simulink library "ODEHubs_components"  (R2020b)
settings: Solver=VariableStepAuto  StartTime=0.0  StopTime=10.0  RelTol=1e-3
values from neighbouring files (symbols this model uses):
  I = aux    [EH_definition_Simulink.m]
  O = aux    [EH_definition_Simulink.m]
undefined symbols (not defined in the file or in its folder): AbsorptionChiller, beta1, BiomassBoiler, Boiler, CN0, CombinedHeatAndPower, cpa, DesalinationPlant, dispatch_factor, DN0, efficiency, HeatPump, IrrigationPump, Low, Low1, Low2, Max_in, Max_out, Min_in, NanofiltrationPlant, PVModules, r_c, r_d, ReversibleHeatPump, SolarCollector, StorageSystem, T_muestreo, Tm, Up, Up1, Up2
(part 2 of 2)

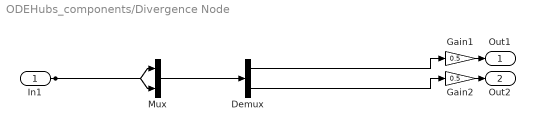
== system ODEHubs_components/Divergence Node ==
  In1 : Inport
  Demux : Demux  Outputs=2
  Gain1 : Gain  Gain=0.5
  Gain2 : Gain  Gain=0.5
  Mux : Mux  Inputs=2
  Out1 : Outport
  Out2 : Outport  Port=2
  wires:
  In1/1 -> Mux/1, Mux/2
  Demux/1 -> Gain1/1
  Gain1/1 -> Out1/1
  Demux/2 -> Gain2/1
  Gain2/1 -> Out2/1
  Mux/1 -> Demux/1

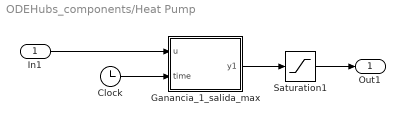
== system ODEHubs_components/Heat Pump ==
  In1 : Inport
  Clock : Clock
  Ganancia_1_salida_max : MATLAB Function  TreatAsAtomicUnit=on  mask{Max_in=10, efficiency=[5.4], T_muestreo=T_muestreo, dispatch_factor=1}
      mask prompts: Max_in "Máximo"; efficiency "Eficiencia"; T_muestreo "Tiempo de muestreo"; dispatch_factor "Coeficiente de reparto"
  Saturation1 : Saturate  UpperLimit=Max_out(1)  LowerLimit=-inf
  Out1 : Outport  VectorParamsAs1DForOutWhenUnconnected=off
  wires:
  Saturation1/1 -> Out1/1
  Clock/1 -> Ganancia_1_salida_max/2(time)
  In1/1 -> Ganancia_1_salida_max/1(u)
  Ganancia_1_salida_max/1(y1) -> Saturation1/1

== system ODEHubs_components/Input ==
  Input : FromWorkspace  VariableName=simin
  Out1 : Outport
  wires:
  Input/1 -> Out1/1

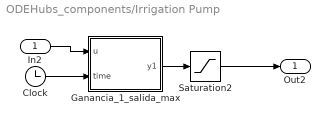
== system ODEHubs_components/Irrigation Pump ==
  In2 : Inport
  Clock : Clock
  Ganancia_1_salida_max : MATLAB Function  TreatAsAtomicUnit=on  mask{Max_in=150, efficiency=1, T_muestreo=T_muestreo, dispatch_factor=beta1}
      mask prompts: Max_in "Máximo"; efficiency "Eficiencia"; T_muestreo "Tiempo de muestreo"; dispatch_factor "Coeficiente de reparto"
  Saturation2 : Saturate  UpperLimit=Max_out  LowerLimit=-inf
  Out2 : Outport  VectorParamsAs1DForOutWhenUnconnected=off
  wires:
  Clock/1 -> Ganancia_1_salida_max/2(time)
  Saturation2/1 -> Out2/1
  In2/1 -> Ganancia_1_salida_max/1(u)
  Ganancia_1_salida_max/1(y1) -> Saturation2/1

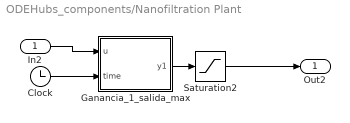
== system ODEHubs_components/Nanofiltration Plant ==
  In2 : Inport
  Clock : Clock
  Ganancia_1_salida_max : MATLAB Function  TreatAsAtomicUnit=on  mask{Max_in=Max_in, efficiency=efficiency, T_muestreo=T_muestreo, dispatch_factor=beta1}
      mask prompts: Max_in "Máximo"; efficiency "Eficiencia"; T_muestreo "Tiempo de muestreo"; dispatch_factor "Coeficiente de reparto"
  Saturation2 : Saturate  UpperLimit=Max_out  LowerLimit=-inf
  Out2 : Outport  VectorParamsAs1DForOutWhenUnconnected=off
  wires:
  Ganancia_1_salida_max/1(y1) -> Saturation2/1
  Saturation2/1 -> Out2/1
  In2/1 -> Ganancia_1_salida_max/1(u)
  Clock/1 -> Ganancia_1_salida_max/2(time)

== system ODEHubs_components/Output ==
  In1 : Inport
  Market Sales : Constant  Value=0
  Output : ToWorkspace  VariableName=simout  SaveFormat=Timeseries  SampleTime=-1
  Sum : Sum  Inputs=-+|
  wires:
  In1/1 -> Sum/2
  Sum/1 -> Output/1
  Market Sales/1 -> Sum/1

== system ODEHubs_components/PV Modules ==
  In1 : Inport
  Clock : Clock
  Ganancia_1_salida_max : MATLAB Function  TreatAsAtomicUnit=on  mask{Max_in=1200, efficiency=[0.211], T_muestreo=T_muestreo, dispatch_factor=1}
      mask prompts: Max_in "Máximo"; efficiency "Eficiencia"; T_muestreo "Tiempo de muestreo"; dispatch_factor "Coeficiente de reparto"
  Saturation1 : Saturate  UpperLimit=Max_out  LowerLimit=-inf
  Out1 : Outport  VectorParamsAs1DForOutWhenUnconnected=off
  wires:
  Saturation1/1 -> Out1/1
  Ganancia_1_salida_max/1(y1) -> Saturation1/1
  In1/1 -> Ganancia_1_salida_max/1(u)
  Clock/1 -> Ganancia_1_salida_max/2(time)

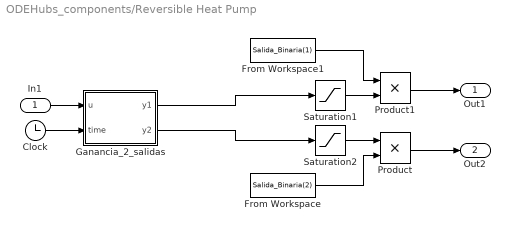
== system ODEHubs_components/Reversible Heat Pump ==
  In1 : Inport
  Clock : Clock
  From Workspace : FromWorkspace  VariableName=Salida_Binaria(2)
  From Workspace1 : FromWorkspace  VariableName=Salida_Binaria(1)
  Ganancia_2_salidas : MATLAB Function  TreatAsAtomicUnit=on  mask{efficiency=efficiency, T_muestreo=T_muestreo, Max_in=Max_in, Min_in=Min_in, dispatch_factor=1}
      mask prompts: efficiency "Eficiencia"; T_muestreo "Tiempo de muestreo"; Max_in "Entrada máxima"; Min_in "Entrada mínima"; dispatch_factor "Coeficiente de reparto"
  Product : Product
  Product1 : Product
  Saturation1 : Saturate  UpperLimit=Max_out(1)  LowerLimit=-inf
  Saturation2 : Saturate  UpperLimit=Max_out(2)  LowerLimit=-inf
  Out1 : Outport  VectorParamsAs1DForOutWhenUnconnected=off
  Out2 : Outport  Port=2  VectorParamsAs1DForOutWhenUnconnected=off
  wires:
  In1/1 -> Ganancia_2_salidas/1(u)
  Clock/1 -> Ganancia_2_salidas/2(time)
  Ganancia_2_salidas/1(y1) -> Saturation1/1
  Ganancia_2_salidas/2(y2) -> Saturation2/1
  Product/1 -> Out2/1
  Saturation2/1 -> Product/1
  Saturation1/1 -> Product1/2
  Product1/1 -> Out1/1
  From Workspace/1 -> Product/2
  From Workspace1/1 -> Product1/1

== system ODEHubs_components/Solar Collector ==
  In1 : Inport
  Clock : Clock
  Ganancia_1_salida_max : MATLAB Function  TreatAsAtomicUnit=on  mask{Max_in=1200, efficiency=[0.211], T_muestreo=T_muestreo, dispatch_factor=1}
      mask prompts: Max_in "Máximo"; efficiency "Eficiencia"; T_muestreo "Tiempo de muestreo"; dispatch_factor "Coeficiente de reparto"
  Saturation1 : Saturate  UpperLimit=Max_out  LowerLimit=-inf
  Out1 : Outport  VectorParamsAs1DForOutWhenUnconnected=off
  wires:
  In1/1 -> Ganancia_1_salida_max/1(u)
  Clock/1 -> Ganancia_1_salida_max/2(time)
  Ganancia_1_salida_max/1(y1) -> Saturation1/1
  Saturation1/1 -> Out1/1

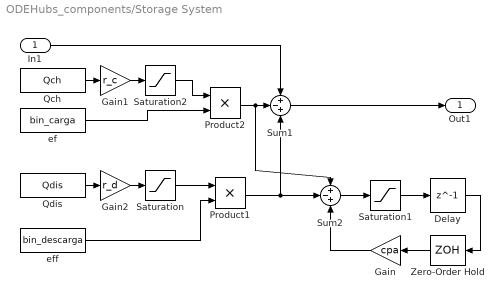
== system ODEHubs_components/Storage System ==
  In1 : Inport
  Delay : Delay  DelayLength=1  InitialCondition=0
  Gain : Gain  Gain=cpa
  Gain1 : Gain  Gain=r_c
  Gain2 : Gain  Gain=r_d
  Product1 : Product
  Product2 : Product
  Qch : FromWorkspace  VariableName=Qch  SampleTime=-1
  Qdis : FromWorkspace  VariableName=Qdis  SampleTime=-1
  Saturation : Saturate  UpperLimit=Up  LowerLimit=Low
  Saturation1 : Saturate  UpperLimit=Up1  LowerLimit=Low1
  Saturation2 : Saturate  UpperLimit=Up2  LowerLimit=Low2
  Sum1 : Sum  Inputs=+-+
  Sum2 : Sum  Inputs=+-+
  Zero-Order Hold : ZeroOrderHold  SampleTime=-1
  ef : FromWorkspace  VariableName=bin_carga  SampleTime=-1
  eff : FromWorkspace  VariableName=bin_descarga  SampleTime=-1
  Out1 : Outport  VectorParamsAs1DForOutWhenUnconnected=off
  wires:
  Qdis/1 -> Gain2/1
  ef/1 -> Product2/2
  eff/1 -> Product1/2
  Saturation1/1 -> Delay/1
  In1/1 -> Sum1/1
  Sum1/1 -> Out1/1
  Sum2/1 -> Saturation1/1
  Delay/1 -> Zero-Order Hold/1
  Zero-Order Hold/1 -> Gain/1
  Gain/1 -> Sum2/3
  Qch/1 -> Gain1/1
  Gain1/1 -> Saturation2/1
  Gain2/1 -> Saturation/1
  Saturation/1 -> Product1/1
  Product1/1 -> Sum2/2, Sum1/3
  Saturation2/1 -> Product2/1
  Product2/1 -> Sum2/1, Sum1/2

== matlab function ODEHubs_components/Biomass Boiler/Ganancia_2_salidas ==
  data: u input; y1 output; time input; y2 output; Min_in parameter; Max_in parameter; efficiency parameter; T_muestreo parameter; dispatch_factor parameter
function [y1,y2] = fcn(u,time, Min_in, Max_in, efficiency, T_muestreo, dispatch_factor)

%efficiency: eficiencia
%Max_in: límite de entrada superior
%Min_in: límite de entrada inferior
%T_muestreo: tiempo de muestreo
%dispatch_factor: coeficiente de reparto
%time: tiempo de simulación
%u: entrada
%y1: salida 1
%y2: salida 2

g=efficiency;
if(size(dispatch_factor,2)>1||size(g,1)>1)
    aux=floor(time/T_muestreo)+1;
    if(size(g,1)==1)
        u = max_min_u(u,dispatch_factor(aux),Min_in, Max_in);
        y1=u*dispatch_factor(aux)*g(1,1);
        y2=u*dispatch_factor(aux)*g(1,2);
    end
    if(size(dispatch_factor,2)==1)
        u = max_min_u(u,dispatch_factor, Min_in, Max_in);
        y1=u*dispatch_factor*g(aux,1);
        y2=u*dispatch_factor*g(aux,2);
    end
else
    u = max_min_u(u,dispatch_factor ,Min_in, Max_in);
    y1=u*dispatch_factor*g(1,1);
    y2=u*dispatch_factor*g(1,2);
end

end

% obtengo los límites de entrada de energía del dispositivo
function u = max_min_u(a,dispatch_factor, Min_in, Max_in)
if(a*dispatch_factor>Max_in)
    u=Max_in;
else
    u=a;
end
if(a*dispatch_factor<Min_in)
    u=Min_in;
else
    u=a;
end
end

== matlab function ODEHubs_components/PV Modules/Ganancia_1_salida_max ==
  data: u input; y1 output; time input; dispatch_factor parameter; T_muestreo parameter; efficiency parameter; Max_in parameter
function y1  = fcn(u,time, dispatch_factor, T_muestreo, efficiency, Max_in)
%efficiency: eficiencia
%Max_in: límite de entrada superior
%T_muestreo: tiempo de muestreo
%dispatch_factor: coeficiente de reparto
%time: tiempo de simulación
%u: entrada
%y1:salida

g=efficiency;

if(size(dispatch_factor,2)>1||size(g,1)>1)
    aux=floor(time/T_muestreo)+1;
    if(size(g,1)==1)
        u = max_min_u(u,dispatch_factor(aux), Max_in);
        y1=u*dispatch_factor(aux)*g;
    end
    if(size(dispatch_factor,2)==1)
        u = max_min_u(u,dispatch_factor,Max_in);
        y1=u*dispatch_factor*g(aux);
    end
else
    u = max_min_u(u,dispatch_factor,Max_in);
    y1=u*dispatch_factor*g;
end
end

% obtengo los límites de entrada de energía del dispositivo
function u = max_min_u(a,dispatch_factor,Max_in)
if(a*dispatch_factor>Max_in)
    u=Max_in;
else
    u=a;
end
end

== matlab function ODEHubs_components/Desalination Plant/Ganancia_1_salida_max ==
  data: u input; y1 output; time input; dispatch_factor parameter; T_muestreo parameter; efficiency parameter; Max_in parameter
function y1  = fcn(u,time, dispatch_factor, T_muestreo, efficiency, Max_in)
g=efficiency;

if(size(dispatch_factor,2)>1||size(g,1)>1)
    aux=floor(time/T_muestreo)+1;
    if(size(g,1)==1)
        u = max_min_u(u,dispatch_factor(aux), Max_in);
        y1=u*dispatch_factor(aux)*g;
    end
    if(size(dispatch_factor,2)==1)
        u = max_min_u(u,dispatch_factor,Max_in);
        y1=u*dispatch_factor*g(aux);
    end
else
    u = max_min_u(u,dispatch_factor,Max_in);
    y1=u*dispatch_factor*g;
end
end

% obtengo los límites de entrada de energía del dispositivo
function u = max_min_u(a,dispatch_factor,Max_in)
if(a*dispatch_factor>Max_in)
    u=Max_in;
else
    u=a;
end
end

== matlab function ODEHubs_components/Boiler/Ganancia_1_salida_max_min ==
  data: u input; y1 output; time input; Min_in parameter; Max_in parameter; efficiency parameter; T_muestreo parameter; dispatch_factor parameter
function y1  = fcn(u,time, Min_in, Max_in, efficiency, T_muestreo, dispatch_factor)
%efficiency: eficiencia
%Max_in: límite de entrada superior
%Min_in: límite de entrada inferior
%T_muestreo: tiempo de muestreo
%dispatch_factor: coeficiente de reparto
%time: tiempo de simulación
%u: entrada
%y1:salida
g=efficiency;
if(size(dispatch_factor,2)>1||size(g,1)>1)
    aux=floor(time/T_muestreo)+1;
    if(size(g,1)==1)
        u=min_max(u,dispatch_factor(aux),Max_in,Min_in)
        y1=u*dispatch_factor(aux)*g;
    end
    if(size(dispatch_factor,2)==1)
        u=min_max(u,dispatch_factor,Max_in,Min_in)
        y1=u*dispatch_factor*g(aux);
    end
else
    u=min_max(u,dispatch_factor,Max_in,Min_in)
    y1=u*dispatch_factor*g;
end
end

%obtengo los límites de entrada al dispositivo
function u=min_max(a,dispatch_factor,Max_in,Min_in)
if(a*dispatch_factor>Max_in)
    u=Max_in;
else
    u=a;
end
if(a*dispatch_factor<Min_in)
    u=Min_in;
else
    u=a;
end
end

== matlab function ODEHubs_components/Solar Collector/Ganancia_1_salida_max ==
  data: u input; y1 output; time input; dispatch_factor parameter; T_muestreo parameter; efficiency parameter; Max_in parameter
function y1  = fcn(u,time, dispatch_factor, T_muestreo, efficiency, Max_in)
%efficiency: eficiencia
%Max_in: límite de entrada superior
%T_muestreo: tiempo de muestreo
%dispatch_factor: coeficiente de reparto
%time: tiempo de simulación
%u: entrada
%y1:salida

g=efficiency;

if(size(dispatch_factor,2)>1||size(g,1)>1)
    aux=floor(time/T_muestreo)+1;
    if(size(g,1)==1)
        u = max_min_u(u,dispatch_factor(aux), Max_in);
        y1=u*dispatch_factor(aux)*g;
    end
    if(size(dispatch_factor,2)==1)
        u = max_min_u(u,dispatch_factor,Max_in);
        y1=u*dispatch_factor*g(aux);
    end
else
    u = max_min_u(u,dispatch_factor,Max_in);
    y1=u*dispatch_factor*g;
end
end

% obtengo los límites de entrada de energía del dispositivo
function u = max_min_u(a,dispatch_factor,Max_in)
if(a*dispatch_factor>Max_in)
    u=Max_in;
else
    u=a;
end
end

== matlab function ODEHubs_components/Combined Heat and Power/Ganancia_2_salidas ==
  data: u input; y1 output; time input; y2 output; Min_in parameter; Max_in parameter; efficiency parameter; T_muestreo parameter; dispatch_factor parameter
function [y1,y2] = fcn(u,time, Min_in, Max_in, efficiency, T_muestreo, dispatch_factor)

%efficiency: eficiencia
%Max_in: límite de entrada superior
%Min_in: límite de entrada inferior
%T_muestreo: tiempo de muestreo
%dispatch_factor: coeficiente de reparto
%time: tiempo de simulación
%u: entrada
%y1: salida 1
%y2: salida 2

g=efficiency;
if(size(dispatch_factor,2)>1||size(g,1)>1)
    aux=floor(time/T_muestreo)+1;
    if(size(g,1)==1)
        u = max_min_u(u,dispatch_factor(aux),Min_in, Max_in);
        y1=u*dispatch_factor(aux)*g(1,1);
        y2=u*dispatch_factor(aux)*g(1,2);
    end
    if(size(dispatch_factor,2)==1)
        u = max_min_u(u,dispatch_factor, Min_in, Max_in);
        y1=u*dispatch_factor*g(aux,1);
        y2=u*dispatch_factor*g(aux,2);
    end
else
    u = max_min_u(u,dispatch_factor ,Min_in, Max_in);
    y1=u*dispatch_factor*g(1,1);
    y2=u*dispatch_factor*g(1,2);
end

end

% obtengo los límites de entrada de energía del dispositivo
function u = max_min_u(a,dispatch_factor, Min_in, Max_in)
if(a*dispatch_factor>Max_in)
    u=Max_in;
else
    u=a;
end
if(a*dispatch_factor<Min_in)
    u=Min_in;
else
    u=a;
end
end

== matlab function ODEHubs_components/Heat Pump/Ganancia_1_salida_max ==
  data: u input; y1 output; time input; dispatch_factor parameter; T_muestreo parameter; efficiency parameter; Max_in parameter
function y1  = fcn(u,time, dispatch_factor, T_muestreo, efficiency, Max_in)
g=efficiency;

if(size(dispatch_factor,2)>1||size(g,1)>1)
    aux=floor(time/T_muestreo)+1;
    if(size(g,1)==1)
        u = max_min_u(u,dispatch_factor(aux), Max_in);
        y1=u*dispatch_factor(aux)*g;
    end
    if(size(dispatch_factor,2)==1)
        u = max_min_u(u,dispatch_factor,Max_in);
        y1=u*dispatch_factor*g(aux);
    end
else
    u = max_min_u(u,dispatch_factor,Max_in);
    y1=u*dispatch_factor*g;
end
end

% obtengo los límites de entrada de energía del dispositivo
function u = max_min_u(a,dispatch_factor,Max_in)
if(a*dispatch_factor>Max_in)
    u=Max_in;
else
    u=a;
end
end

== matlab function ODEHubs_components/Absorption Chiller/Ganancia_1_salida_max_min ==
  data: u input; y1 output; time input; Min_in parameter; Max_in parameter; efficiency parameter; T_muestreo parameter; dispatch_factor parameter
function y1  = fcn(u,time, Min_in, Max_in, efficiency, T_muestreo, dispatch_factor)
g=efficiency;
if(size(dispatch_factor,2)>1||size(g,1)>1)
    aux=floor(time/T_muestreo)+1;
    if(size(g,1)==1)
        u=min_max(u,dispatch_factor(aux),Max_in,Min_in)
        y1=u*dispatch_factor(aux)*g;
    end
    if(size(dispatch_factor,2)==1)
        u=min_max(u,dispatch_factor,Max_in,Min_in)
        y1=u*dispatch_factor*g(aux);
    end
else
    u=min_max(u,dispatch_factor,Max_in,Min_in)
    y1=u*dispatch_factor*g;
end
end

%obtengo los límites de entrada al dispositivo
function u=min_max(a,dispatch_factor,Max_in,Min_in)
if(a*dispatch_factor>Max_in)
    u=Max_in;
else
    u=a;
end
if(a*dispatch_factor<Min_in)
    u=Min_in;
else
    u=a;
end
end

== matlab function ODEHubs_components/Reversible Heat Pump/Ganancia_2_salidas ==
  data: u input; y1 output; time input; y2 output; Min_in parameter; Max_in parameter; efficiency parameter; T_muestreo parameter; dispatch_factor parameter
function [y1,y2] = fcn(u,time, Min_in, Max_in, efficiency, T_muestreo, dispatch_factor)
g=efficiency;
if(size(dispatch_factor,2)>1||size(g,1)>1)
    aux=floor(time/T_muestreo)+1;
    if(size(g,1)==1)
        u = max_min_u(u,dispatch_factor(aux),Min_in, Max_in);
        y1=u*dispatch_factor(aux)*g(1,1);
        y2=u*dispatch_factor(aux)*g(1,2);
    end
    if(size(dispatch_factor,2)==1)
        u = max_min_u(u,dispatch_factor, Min_in, Max_in);
        y1=u*dispatch_factor*g(aux,1);
        y2=u*dispatch_factor*g(aux,2);
    end
else
    u = max_min_u(u,dispatch_factor ,Min_in, Max_in);
    y1=u*dispatch_factor*g(1,1);
    y2=u*dispatch_factor*g(1,2);
end

end

% obtengo los límites de entrada de energía del dispositivo
function u = max_min_u(a,dispatch_factor, Min_in, Max_in)
if(a*dispatch_factor>Max_in)
    u=Max_in;
else
    u=a;
end
if(a*dispatch_factor<Min_in)
    u=Min_in;
else
    u=a;
end
end

== matlab function ODEHubs_components/Nanofiltration Plant/Ganancia_1_salida_max ==
  data: u input; y1 output; time input; dispatch_factor parameter; T_muestreo parameter; efficiency parameter; Max_in parameter
function y1  = fcn(u,time, dispatch_factor, T_muestreo, efficiency, Max_in)
g=efficiency;

if(size(dispatch_factor,2)>1||size(g,1)>1)
    aux=floor(time/T_muestreo)+1;
    if(size(g,1)==1)
        u = max_min_u(u,dispatch_factor(aux), Max_in);
        y1=u*dispatch_factor(aux)*g;
    end
    if(size(dispatch_factor,2)==1)
        u = max_min_u(u,dispatch_factor,Max_in);
        y1=u*dispatch_factor*g(aux);
    end
else
    u = max_min_u(u,dispatch_factor,Max_in);
    y1=u*dispatch_factor*g;
end
end

% obtengo los límites de entrada de energía del dispositivo
function u = max_min_u(a,dispatch_factor,Max_in)
if(a*dispatch_factor>Max_in)
    u=Max_in;
else
    u=a;
end
end

== matlab function ODEHubs_components/Irrigation Pump/Ganancia_1_salida_max ==
  data: u input; y1 output; time input; dispatch_factor parameter; T_muestreo parameter; efficiency parameter; Max_in parameter
function y1  = fcn(u,time, dispatch_factor, T_muestreo, efficiency, Max_in)
g=efficiency;

if(size(dispatch_factor,2)>1||size(g,1)>1)
    aux=floor(time/T_muestreo)+1;
    if(size(g,1)==1)
        u = max_min_u(u,dispatch_factor(aux), Max_in);
        y1=u*dispatch_factor(aux)*g;
    end
    if(size(dispatch_factor,2)==1)
        u = max_min_u(u,dispatch_factor,Max_in);
        y1=u*dispatch_factor*g(aux);
    end
else
    u = max_min_u(u,dispatch_factor,Max_in);
    y1=u*dispatch_factor*g;
end
end

% obtengo los límites de entrada de energía del dispositivo
function u = max_min_u(a,dispatch_factor,Max_in)
if(a*dispatch_factor>Max_in)
    u=Max_in;
else
    u=a;
end
end
